simulink model "PlantARMAX"  (R2020b)
settings: Solver=ode45  StartTime=0.0  StopTime=Tend  RelTol=1e-3  EnableMultiTasking=on
values from neighbouring files (symbols this model uses):
  c10 = 0.7    [init2.m]
  Td = 100    [init2.m]
  Tp = 0.1    [init2.m]
libraries: simulink x1
settings Model: Creator=Melkamu A  LastModifiedBy=Melkamu A
settings DataIOCC: SaveFormat=Array  SignalLoggingSaveFormat=ModelDataLogs  ReturnWorkspaceOutputs=off
settings OptimizationCC: InitFltsAndDblsToZero=on  LifeSpan=inf
settings DebuggingCC: SaveWithParameterizedLinksMsg=none  UnderspecifiedInitializationDetection=Classic  MergeDetectMultiDrivingBlocksExec=none  SignalResolutionControl=TryResolveAllWithWarning  SolverPrmCheckMsg=warning  MultiTaskDSMMsg=warning  MultiTaskCondExecSysMsg=none  FcnCallInpInsideContextMsg=warning  SFUnexpectedBacktrackingDiag=warning  SFNoUnconditionalDefaultTransitionDiag=warning  SFExecutionAtInitializationDiag=none  ArithmeticOperatorsInVariantConditions=warning
settings HardwareCC: ProdBitPerPointer=32  ProdBitPerSizeT=32  ProdBitPerPtrDiffT=32  ProdLargestAtomicFloat=None  ProdIntDivRoundTo=Undefined  ProdEndianess=Unspecified  ProdWordSize=32  ProdHWDeviceType=32-bit Generic
settings ModelReferenceCC: PropagateSignalLabelsOutOfModel=off
settings CodeAppCC: StateflowObjectComments=on
settings GRTTargetCC: TargetFcnLib=ansi_tfl_tmw.mat  TargetLangStandard=C89/C90 (ANSI)  CombineOutputUpdateFcns=off  GRTInterface=on
settings ConfigComp: CovMetricSettings=dw  CovSaveCumulativeToWorkspaceVar=on  CovSaveSingleToWorkspaceVar=on

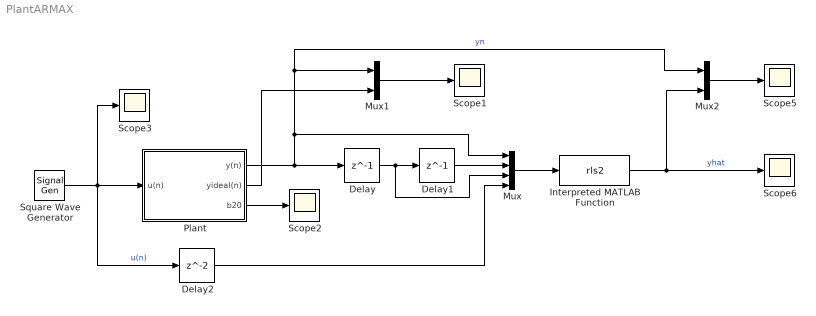
== system PlantARMAX ==
  Delay : Delay  DelayLength=1  SampleTime=Tp
  Delay1 : Delay  DelayLength=1  SampleTime=Tp
  Delay2 : Delay  SampleTime=Tp
  Interpreted MATLAB Function : MATLABFcn  MATLABFcn=rls2
  Mux : Mux
  Mux1 : Mux  Inputs=2
  Mux2 : Mux  Inputs=2
  Plant : Subsystem
  Scope{1..3,5..6} (5 alike) : Scope
  Square Wave Generator : SignalGenerator  WaveForm=square  Frequency=0.2
  wires:
  Delay/1 -> Mux/3, Delay1/1
  Delay1/1 -> Mux/2
  Plant/1(y(n)) -> Mux2/1, Mux1/1, Mux/1, Delay/1  "yn"
  Mux1/1 -> Scope1/1
  Plant/2(yideal(n)) -> Mux1/2
  Plant/3(b20) -> Scope2/1
  Square Wave Generator/1 -> Delay2/1, Scope3/1, Plant/1(u(n))  "u(n)"
  Interpreted MATLAB Function/1 -> Scope6/1, Mux2/2  "yhat"
  Mux2/1 -> Scope5/1
  Mux/1 -> Interpreted MATLAB Function/1
  Delay2/1 -> Mux/4

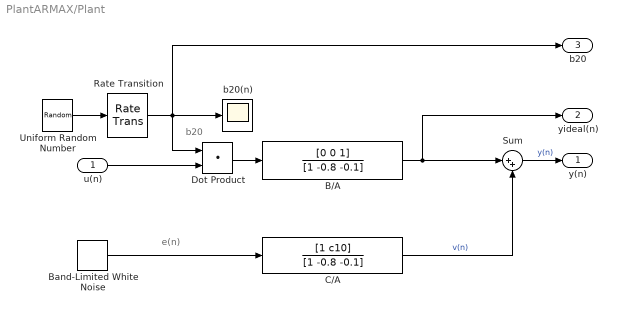
== system PlantARMAX/Plant ==
  note: b20
  note: e(n)
  u(n) : Inport
  B/A : DiscreteFilter  Numerator=[0 0 1]  Denominator=[1 -0.8 -0.1]  SampleTime=Tp
  Band-Limited White Noise : simulink/Sources/Band-Limited White Noise  Cov=[0.01]*Tp  Ts=Tp  seed=[23341]
  C/A : DiscreteFilter  Numerator=[1 c10]  Denominator=[1 -0.8 -0.1]  SampleTime=Tp
  Dot Product : DotProduct  InputSameDT=on  OutDataTypeStr=Inherit: Inherit via internal rule
  Rate Transition : RateTransition  InitialCondition=0.5  OutPortSampleTime=Tp
  Sum : Sum  Inputs=|++  SaturateOnIntegerOverflow=on
  Uniform Random Number : UniformRandomNumber  Minimum=0  Maximum=0.5  SampleTime=Td
  b20(n) : Scope
  y(n) : Outport
  yideal(n) : Outport  Port=2
  b20 : Outport  Port=3
  wires:
  C/A/1 -> Sum/2  "v(n)"
  Sum/1 -> y(n)/1  "y(n)"
  Band-Limited White Noise/1 -> C/A/1
  B/A/1 -> yideal(n)/1, Sum/1
  u(n)/1 -> Dot Product/2
  Dot Product/1 -> B/A/1
  Uniform Random Number/1 -> Rate Transition/1
  Rate Transition/1 -> Dot Product/1, b20(n)/1, b20/1
